simulink model "closeLoopv2"  (R2024a)
settings: Solver=ode4  StartTime=0.0  StopTime=1000  FixedStep=1E-4  MinStep=1E-4  RelTol=1e-3
values from neighbouring files (symbols this model uses):
  x = [input(1);input(2);input(3)]    [Dist_observer.m]
  y = [input(4),input(5),input(6)]'    [controller.m]
undefined symbols (not defined in the file or in its folder): initial_1, observer, z
settings Model: Creator=b_ant  LastModifiedBy=b_ant
settings SolverCC: InitialStep=1E-4  ZeroCrossAlgorithm=Adaptive
settings DebuggingCC: IgnoredZcDiagnostic=none

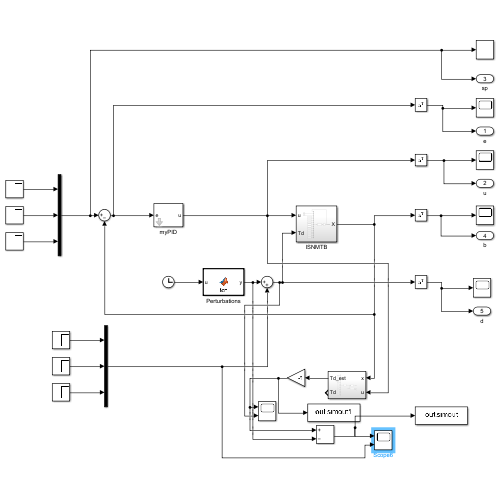
[thumbnail: Simulink's stored preview of the top-level diagram]
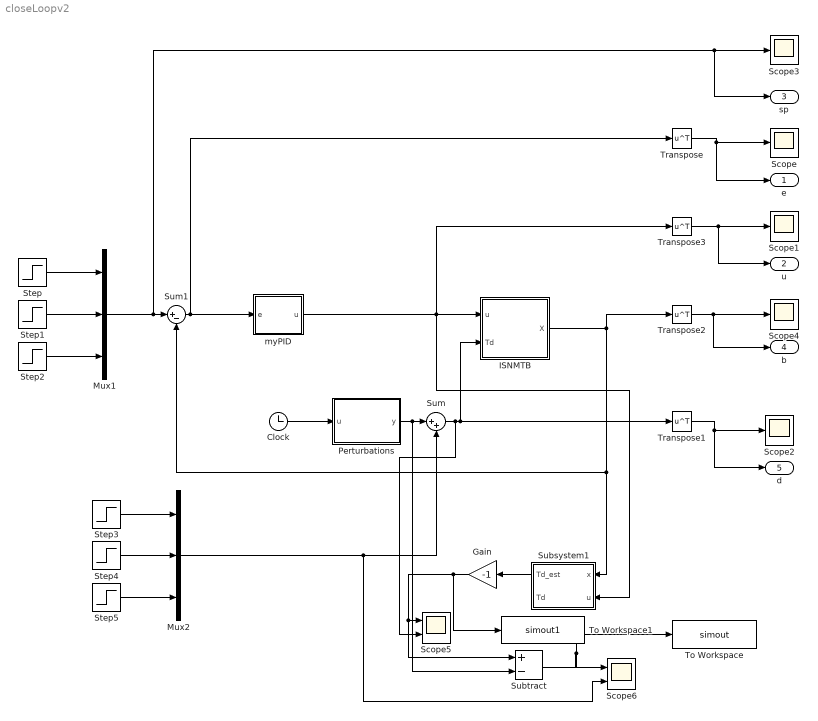
== system closeLoopv2 ==
  Clock : Clock
      settings: Decimation=1000
  Gain : Gain  Gain=-1
  ISNMTB : Subsystem
  Mux1 : Mux  Inputs=3
  Mux2 : Mux  Inputs=3
  Perturbations : MATLAB Function  TreatAsAtomicUnit=on
  Scope{,1..4} (5 alike) : Scope
  Scope5 : Scope  NumInputPorts=2
  Scope6 : Scope  NumInputPorts=2
  Step : Step  Time=0.1  After=0  SampleTime=0
  Step1 : Step  Time=0.1  After=0  SampleTime=0
  Step2 : Step  Time=0.1  After=0  SampleTime=0
  Step3 : Step  Time=5  After=10  SampleTime=0
  Step4 : Step  Time=5  After=20  SampleTime=0
  Step5 : Step  Time=5  After=30  SampleTime=0
  Subsystem1 : Subsystem
  Subtract : Sum  Inputs=+-
  Sum : Sum  Inputs=|++
  Sum1 : Sum  Inputs=|+-
  To Workspace : ToWorkspace  VariableName=simout  SampleTime=-1
  To Workspace1 : ToWorkspace  VariableName=simout1  SampleTime=-1
  Transpose{,1..3} (4 alike) : Math  Operator=transpose
  myPID : Subsystem
  e : Outport
  u : Outport  Port=2
  sp : Outport  Port=3
  b : Outport  Port=4
  d : Outport  Port=5
  wires:
  Step2/1 -> Mux1/3
  Sum1/1 -> myPID/1(e), Transpose/1
  Step1/1 -> Mux1/2
  Clock/1 -> Perturbations/1(u)
  Step/1 -> Mux1/1
  Transpose/1 -> e/1, Scope/1
  Transpose1/1 -> Scope2/1, d/1
  ISNMTB/1(X) -> Transpose2/1, Subsystem1/1(x), Sum1/2
  Transpose2/1 -> b/1, Scope4/1
  Transpose3/1 -> u/1, Scope1/1
  Mux1/1 -> sp/1, Scope3/1, Sum1/1
  myPID/1(u) -> Subsystem1/2(u), Transpose3/1, ISNMTB/1(u)
  Step3/1 -> Mux2/1
  Step4/1 -> Mux2/2
  Step5/1 -> Mux2/3
  Perturbations/1(y) -> Subtract/2, Sum/1
  Sum/1 -> Scope5/2, ISNMTB/2(Td), Transpose1/1
  Mux2/1 -> Scope6/2, Sum/2
  Subsystem1/1(Td_est) -> Gain/1
  Gain/1 -> To Workspace1/1, Subtract/1, Scope5/1
  Subtract/1 -> To Workspace/1, Scope6/1

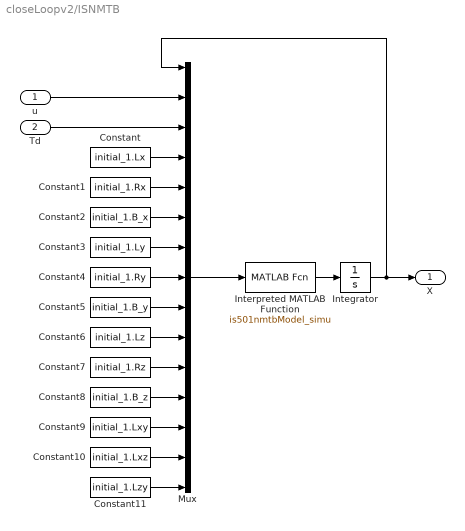
== system closeLoopv2/ISNMTB ==
  u : Inport
  Td : Inport  Port=2
  Constant : Constant  Value=initial_1.Lx
  Constant1 : Constant  Value=initial_1.Rx
  Constant10 : Constant  Value=initial_1.Lxz
  Constant11 : Constant  Value=initial_1.Lzy
  Constant2 : Constant  Value=initial_1.B_x
  Constant3 : Constant  Value=initial_1.Ly
  Constant4 : Constant  Value=initial_1.Ry
  Constant5 : Constant  Value=initial_1.B_y
  Constant6 : Constant  Value=initial_1.Lz
  Constant7 : Constant  Value=initial_1.Rz
  Constant8 : Constant  Value=initial_1.B_z
  Constant9 : Constant  Value=initial_1.Lxy
  Integrator : Integrator  InitialCondition=[3.249E4, -2.265E4, 3.655E4]
  Interpreted MATLAB Function : MATLABFcn  MATLABFcn=is501nmtbModel_simu
  Mux : Mux  Inputs=15
  X : Outport
  wires:
  Interpreted MATLAB Function/1 -> Integrator/1
  Integrator/1 -> X/1, Mux/1
  Mux/1 -> Interpreted MATLAB Function/1
  u/1 -> Mux/2
  Td/1 -> Mux/3
  Constant/1 -> Mux/4
  Constant1/1 -> Mux/5
  Constant2/1 -> Mux/6
  Constant3/1 -> Mux/7
  Constant4/1 -> Mux/8
  Constant5/1 -> Mux/9
  Constant6/1 -> Mux/10
  Constant7/1 -> Mux/11
  Constant8/1 -> Mux/12
  Constant9/1 -> Mux/13
  Constant10/1 -> Mux/14
  Constant11/1 -> Mux/15

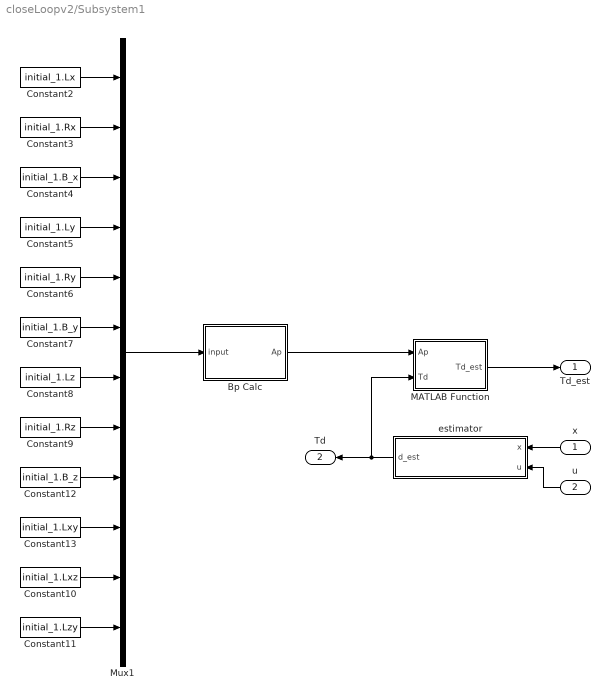
== system closeLoopv2/Subsystem1 ==
  x : Inport
  u : Inport  Port=2
  Bp Calc : MATLAB Function  TreatAsAtomicUnit=on
  Constant10 : Constant  Value=initial_1.Lxz
  Constant11 : Constant  Value=initial_1.Lzy
  Constant12 : Constant  Value=initial_1.B_z
  Constant13 : Constant  Value=initial_1.Lxy
  Constant2 : Constant  Value=initial_1.Lx
  Constant3 : Constant  Value=initial_1.Rx
  Constant4 : Constant  Value=initial_1.B_x
  Constant5 : Constant  Value=initial_1.Ly
  Constant6 : Constant  Value=initial_1.Ry
  Constant7 : Constant  Value=initial_1.B_y
  Constant8 : Constant  Value=initial_1.Lz
  Constant9 : Constant  Value=initial_1.Rz
  MATLAB Function : MATLAB Function  TreatAsAtomicUnit=on
  Mux1 : Mux  Inputs=12
  estimator : Subsystem
  Td_est : Outport
  Td : Outport  Port=2
  wires:
  Constant6/1 -> Mux1/5
  Constant4/1 -> Mux1/3
  estimator/1(d_est) -> Td/1, MATLAB Function/2(Td)
  Constant2/1 -> Mux1/1
  Constant10/1 -> Mux1/11
  Constant13/1 -> Mux1/10
  Constant5/1 -> Mux1/4
  Constant12/1 -> Mux1/9
  Constant3/1 -> Mux1/2
  Constant9/1 -> Mux1/8
  Mux1/1 -> Bp Calc/1(input)
  Constant7/1 -> Mux1/6
  Constant8/1 -> Mux1/7
  Constant11/1 -> Mux1/12
  Bp Calc/1(Ap) -> MATLAB Function/1(Ap)
  x/1 -> estimator/1(x)
  MATLAB Function/1(Td_est) -> Td_est/1
  u/1 -> estimator/2(u)

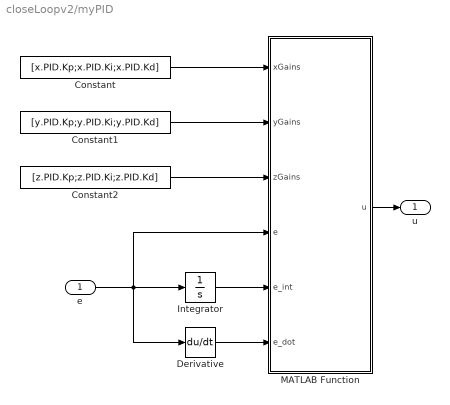
== system closeLoopv2/myPID ==
  e : Inport
  Constant : Constant  Value=[x.PID.Kp;x.PID.Ki;x.PID.Kd]
  Constant1 : Constant  Value=[y.PID.Kp;y.PID.Ki;y.PID.Kd]
  Constant2 : Constant  Value=[z.PID.Kp;z.PID.Ki;z.PID.Kd]
  Derivative : Derivative
  Integrator : Integrator
  MATLAB Function : MATLAB Function  TreatAsAtomicUnit=on
  u : Outport
  wires:
  MATLAB Function/1(u) -> u/1
  e/1 -> Derivative/1, MATLAB Function/4(e), Integrator/1
  Derivative/1 -> MATLAB Function/6(e_dot)
  Integrator/1 -> MATLAB Function/5(e_int)
  Constant1/1 -> MATLAB Function/2(yGains)
  Constant/1 -> MATLAB Function/1(xGains)
  Constant2/1 -> MATLAB Function/3(zGains)

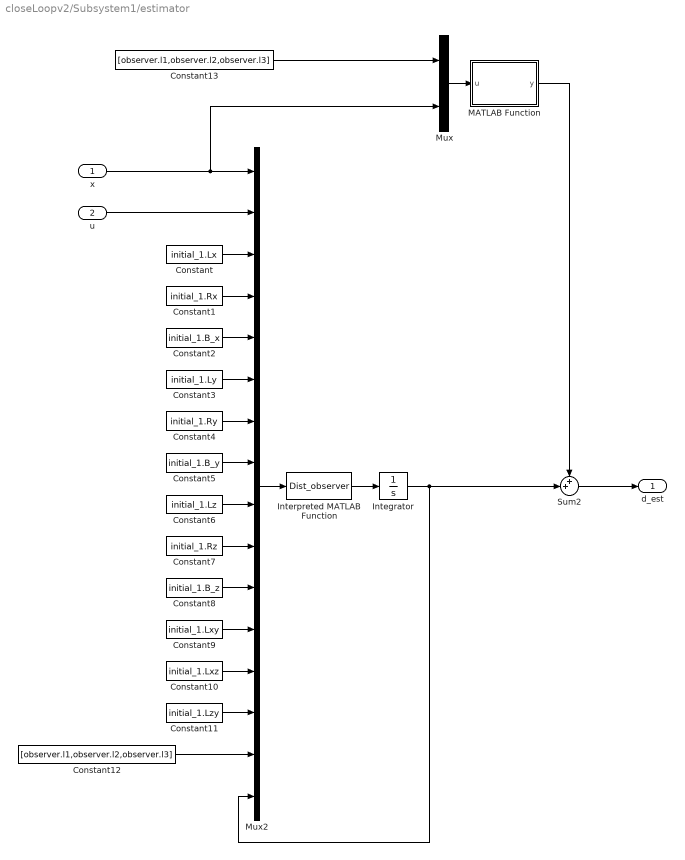
== system closeLoopv2/Subsystem1/estimator ==
  x : Inport
  u : Inport  Port=2
  Constant : Constant  Value=initial_1.Lx
  Constant1 : Constant  Value=initial_1.Rx
  Constant10 : Constant  Value=initial_1.Lxz
  Constant11 : Constant  Value=initial_1.Lzy
  Constant12 : Constant  Value=[observer.l1,observer.l2,observer.l3]
  Constant13 : Constant  Value=[observer.l1,observer.l2,observer.l3]
  Constant2 : Constant  Value=initial_1.B_x
  Constant3 : Constant  Value=initial_1.Ly
  Constant4 : Constant  Value=initial_1.Ry
  Constant5 : Constant  Value=initial_1.B_y
  Constant6 : Constant  Value=initial_1.Lz
  Constant7 : Constant  Value=initial_1.Rz
  Constant8 : Constant  Value=initial_1.B_z
  Constant9 : Constant  Value=initial_1.Lxy
  Integrator : Integrator  InitialCondition=[0,0,0]
  Interpreted MATLAB Function : MATLABFcn  MATLABFcn=Dist_observer
  MATLAB Function : MATLAB Function  TreatAsAtomicUnit=on
  Mux : Mux  Inputs=2
  Mux2 : Mux  Inputs=16
  Sum2 : Sum  Inputs=++|
  d_est : Outport
  wires:
  Constant6/1 -> Mux2/9
  MATLAB Function/1(y) -> Sum2/1
  Constant10/1 -> Mux2/13
  Integrator/1 -> Sum2/2, Mux2/16
  Interpreted MATLAB Function/1 -> Integrator/1
  Constant2/1 -> Mux2/5
  Constant4/1 -> Mux2/7
  Constant7/1 -> Mux2/10
  Mux2/1 -> Interpreted MATLAB Function/1
  Constant11/1 -> Mux2/14
  Constant8/1 -> Mux2/11
  Constant1/1 -> Mux2/4
  Constant3/1 -> Mux2/6
  Constant/1 -> Mux2/3
  Constant9/1 -> Mux2/12
  Constant5/1 -> Mux2/8
  Constant12/1 -> Mux2/15
  u/1 -> Mux2/2
  Sum2/1 -> d_est/1
  Constant13/1 -> Mux/1
  Mux/1 -> MATLAB Function/1(u)
  x/1 -> Mux/2, Mux2/1

== matlab function closeLoopv2/Perturbations ==
  data: u input; y output
function y = fcn(u)
y= [2.522*sin(2*pi*4.788E-3*u)+3.249E04;
   -5.174*sin(2*pi*7.481E-3*u)-2.265E04;
    3.359*sin(2*pi*8.378E-3*u)+3.655E04];
end

== matlab function closeLoopv2/Subsystem1/estimator/MATLAB Function ==
  data: u input; y output
function y = fcn(u)
l = diag([u(1),u(2),u(3)]);
x = [u(4);u(5);u(6)];

y = l*x;
end

== matlab function closeLoopv2/Subsystem1/Bp Calc ==
  data: input input; Ap output
function Ap = fcn(input)
    Lxx =  input(1);
    Rx  =  input(2);
    B_1 =  input(3);
    Lyy =  input(4);
    Ry  =  input(5);
    B_2 =  input(6);
    Lzz =  input(7);
    Rz  =  input(8);
    B_3 =  input(9);
    Lxy =  input(10);
    Lxz =  input(11);
    Lzy =  input(12);

    %%%Parameter reading
    L1 =[Lxx, (B_1/B_2)*Lxy, (B_1/B_3)*Lxz;
        (B_2/B_1)*Lxy, Lyy, (B_2/B_3)*Lzy;
        (B_3/B_1)*Lxz, (B_3/B_2)*Lzy, Lzz];
    L = [Lxx, Lxy, Lxz;
         Lxy, Lyy, Lzy;
         Lxz, Lzy, Lzz];
    R = diag([Rx,Ry,Rz]);
    B = diag([B_1,B_2,B_3]);
    
    %%% Model matrix
    Ap = -inv(L1)*R;
    %Bp =  B*inv(L)*1E9;
    %Bp = Bp';
    %Bp_out = Bp(:);
end

== matlab function closeLoopv2/Subsystem1/MATLAB Function ==
  data: Ap input; Td_est output; Td input
function Td_est = fcn(Ap,Td)
 Td_est = inv(Ap)*Td;
end

== matlab function closeLoopv2/myPID/MATLAB Function ==
  data: xGains input; u output; yGains input; zGains input; e input; e_int input; e_dot input
function u  = Bpid_controller(xGains, yGains, zGains, e, e_int, e_dot) 
    
    kp = diag([xGains(1),yGains(1),zGains(1)]);
    ki = diag([xGains(2),yGains(2),zGains(2)]);
    kd = diag([xGains(3),yGains(3),zGains(3)]);

    u=kp*e+ki*e_int+kd*e_dot;

end
